simulink model "sixdof"  (R2023b)
settings: Solver=VariableStepAuto  StartTime=0.0  StopTime=1  RelTol=1e-3
libraries: shared6dof x5, sharedtransform x4
settings Model: Creator=sphw  LastModifiedBy=sphw

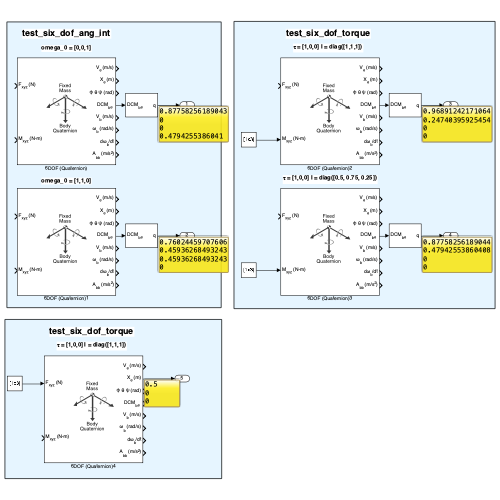
[thumbnail: Simulink's stored preview of the top-level diagram]
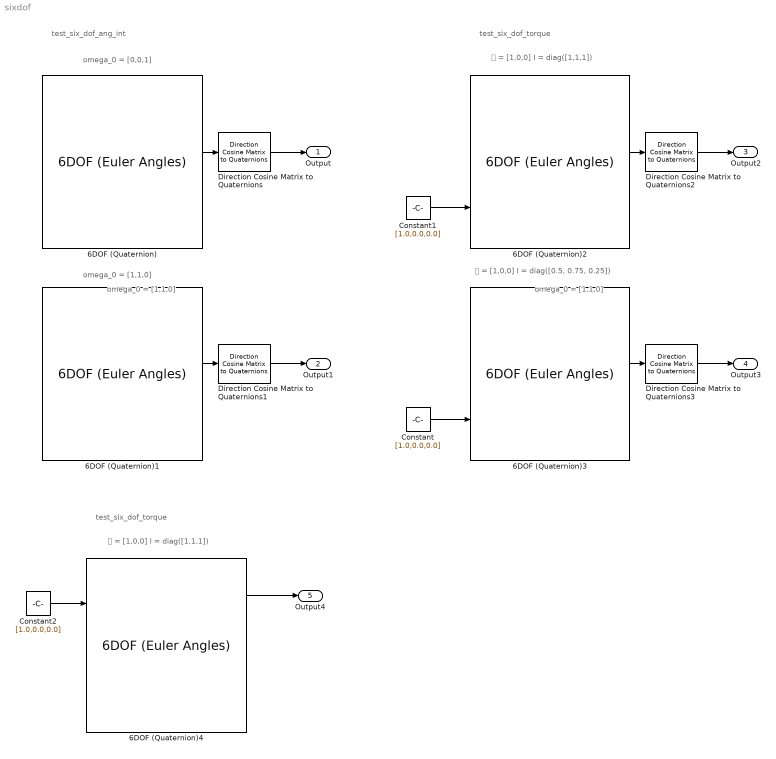
== system sixdof ==
  note: test_six_dof_ang_int
  note: omega_0 = [1,1,0]
  note: omega_0 = [1,1,0]
  note: omega_0 = [0,0,1]
  note: omega_0 = [1,1,0]
  note: 𝛕 = [1,0,0] I = diag([1,1,1])
  note: test_six_dof_torque
  note: 𝛕 = [1,0,0] I = diag([0.5, 0.75, 0.25])
  note: test_six_dof_torque
  note: 𝛕 = [1,0,0] I = diag([1,1,1])
  6DOF (Quaternion) : shared6dof/6DOF (Euler Angles)  units=Metric (MKS)  mtype=Fixed  rep=Quaternion  xme_0=[0 0 0]  Vm_0=[0 0 0]  eul_0=[0 0 0]  pm_0=[0 0 1]  mass_0=1.0  mass_e=0.5  mass_f=2.0  inertia=eye(3)  inertia_e=eye(3)  inertia_f=2*eye(3)  k_quat=1.0  vre_flag=on  abi_flag=off  aMode=0  xme_statename=''  Vm_statename=''  eul_statename=''  quat_statename=''  pm_statename=''  mass_statename=''
      settings: LibrarySourceBlock=aerolib6dof2/6DOF (Quaternion)
  6DOF (Quaternion)1 : shared6dof/6DOF (Euler Angles)  units=Metric (MKS)  mtype=Fixed  rep=Quaternion  xme_0=[0 0 0]  Vm_0=[0 0 0]  eul_0=[0 0 0]  pm_0=[1 1 0]  mass_0=1.0  mass_e=0.5  mass_f=2.0  inertia=eye(3)  inertia_e=eye(3)  inertia_f=2*eye(3)  k_quat=1.0  vre_flag=on  abi_flag=off  aMode=0  xme_statename=''  Vm_statename=''  eul_statename=''  quat_statename=''  pm_statename=''  mass_statename=''
      settings: LibrarySourceBlock=aerolib6dof2/6DOF (Quaternion)
  6DOF (Quaternion)2 : shared6dof/6DOF (Euler Angles)  units=Metric (MKS)  mtype=Fixed  rep=Quaternion  xme_0=[0 0 0]  Vm_0=[0 0 0]  eul_0=[0 0 0]  pm_0=[0 0 0]  mass_0=1.0  mass_e=0.5  mass_f=2.0  inertia=eye(3)  inertia_e=eye(3)  inertia_f=2*eye(3)  k_quat=1.0  vre_flag=on  abi_flag=off  aMode=0  xme_statename=''  Vm_statename=''  eul_statename=''  quat_statename=''  pm_statename=''  mass_statename=''
      settings: LibrarySourceBlock=aerolib6dof2/6DOF (Quaternion)
  6DOF (Quaternion)3 : shared6dof/6DOF (Euler Angles)  units=Metric (MKS)  mtype=Fixed  rep=Quaternion  xme_0=[0 0 0]  Vm_0=[0 0 0]  eul_0=[0 0 0]  pm_0=[0 0 0]  mass_0=1.0  mass_e=0.5  mass_f=2.0  inertia=diag([0.5,0.75,0.25])  inertia_e=eye(3)  inertia_f=2*eye(3)  k_quat=1.0  vre_flag=on  abi_flag=off  aMode=0  xme_statename=''  Vm_statename=''  eul_statename=''  quat_statename=''  pm_statename=''  mass_statename=''
      settings: LibrarySourceBlock=aerolib6dof2/6DOF (Quaternion)
  6DOF (Quaternion)4 : shared6dof/6DOF (Euler Angles)  units=Metric (MKS)  mtype=Fixed  rep=Quaternion  xme_0=[0 0 0]  Vm_0=[0 0 0]  eul_0=[0 0 0]  pm_0=[0 0 0]  mass_0=1.0  mass_e=0.5  mass_f=2.0  inertia=eye(3)  inertia_e=eye(3)  inertia_f=2*eye(3)  k_quat=1.0  vre_flag=on  abi_flag=off  aMode=0  xme_statename=''  Vm_statename=''  eul_statename=''  quat_statename=''  pm_statename=''  mass_statename=''
      settings: LibrarySourceBlock=aerolib6dof2/6DOF (Quaternion)
  Constant : Constant  Value=[1.0,0.0,0.0]  VectorParams1D=off
  Constant1 : Constant  Value=[1.0,0.0,0.0]  VectorParams1D=off
  Constant2 : Constant  Value=[1.0,0.0,0.0]  VectorParams1D=off
  Direction Cosine Matrix to Quaternions{,1..3} (4 alike) : sharedtransform/Direction Cosine Matrix  to Quaternions  aMode=0  action=None  tolerance=eps(2)
      settings: LibrarySourceBlock=|
      | aerolibtransform2/Direction Cosine Matrix
      | to Quaternions
  Output : Outport
  Output1 : Outport  Port=2
  Output2 : Outport  Port=3
  Output3 : Outport  Port=4
  Output4 : Outport  Port=5
  wires:
  Direction Cosine Matrix to Quaternions/1 -> Output/1
  6DOF (Quaternion)/4 -> Direction Cosine Matrix to Quaternions/1
  6DOF (Quaternion)1/4 -> Direction Cosine Matrix to Quaternions1/1
  Direction Cosine Matrix to Quaternions1/1 -> Output1/1
  6DOF (Quaternion)3/4 -> Direction Cosine Matrix to Quaternions3/1
  Direction Cosine Matrix to Quaternions3/1 -> Output3/1
  6DOF (Quaternion)2/4 -> Direction Cosine Matrix to Quaternions2/1
  Direction Cosine Matrix to Quaternions2/1 -> Output2/1
  Constant/1 -> 6DOF (Quaternion)3/2
  Constant1/1 -> 6DOF (Quaternion)2/2
  6DOF (Quaternion)4/2 -> Output4/1
  Constant2/1 -> 6DOF (Quaternion)4/1
